simulink model "sampleModel1922"  (R2023a)
settings: Solver=VariableStepAuto  StartTime=0.0  StopTime=10.0  RelTol=1e-3
libraries: hdlsllib x6, simulink x1
settings Model: Creator=user1  LastModifiedBy=user1

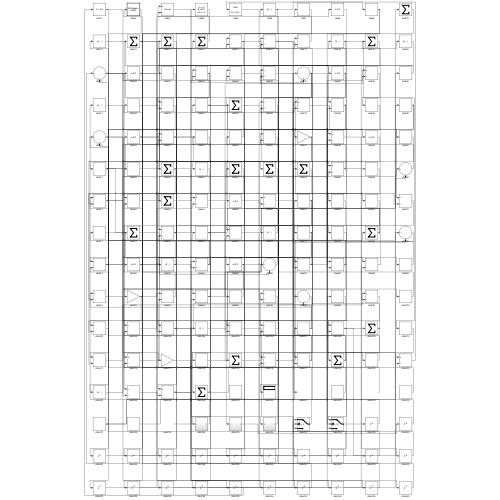
[thumbnail: Simulink's stored preview of the top-level diagram]
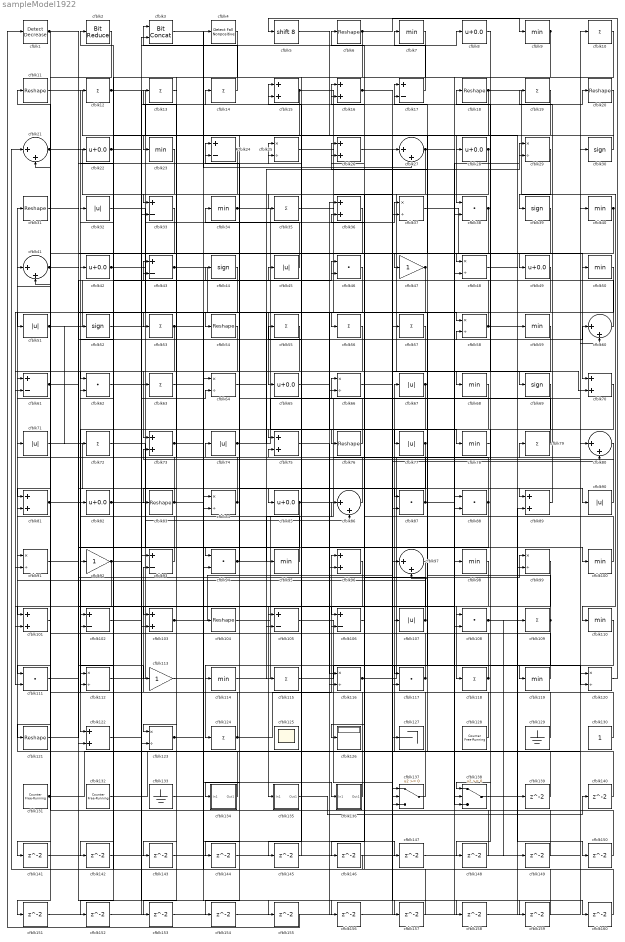
== system sampleModel1922 ==
  cfblk1 : simulink/Logic and Bit Operations/Detect Decrease  vinit=0.0  OutDataTypeStr=boolean
      settings: LibrarySourceBlock=|
      | hdlsllib/Logic and Bit
      | Operations/Detect
      | Decrease
  cfblk{10,12..14,19,35,53,55..57,63,72,79,109,115,118,124} (17 alike) : Sum  Inputs=+
  cfblk{7,9,23,34,40,50,59,68,78,95,98,100,110,114,119} (15 alike) : MinMax
  cfblk{15..16,26,36,70,73,75,81,89,96,101,103,122} (13 alike) : Sum
  cfblk{17,24,33,43,61,93,102,105..106} (9 alike) : Sum  Inputs=+-
  cfblk{6,11,18,20,31,54,76,83,104,121} (10 alike) : Reshape
  cfblk{32,45,51,67,71,74,77,90,107} (9 alike) : Abs  SaturateOnIntegerOverflow=off
  cfblk{38,46,62,87..88,94,108,111,117} (9 alike) : DotProduct  OutDataTypeStr=Inherit: Inherit via internal rule
  cfblk{25,29,37,48,58,64,66,84,91,99,112,116,120,123} (14 alike) : Product  Inputs=*/  RndMeth=Zero  SaturateOnIntegerOverflow=on
  cfblk113 : Gain
  cfblk125 : Scope
      settings: Floating=on
  cfblk126 : Display
  cfblk127 : Terminator
  cfblk128 : hdlsllib/Sources/Counter Free-Running  NumBits=16  tsamp=-1
  cfblk129 : Ground
  cfblk130 : Constant  SampleTime=-1
  cfblk131 : hdlsllib/Sources/Counter Free-Running  NumBits=16  tsamp=-1
  cfblk132 : hdlsllib/Sources/Counter Free-Running  NumBits=16  tsamp=-1
  cfblk133 : Ground
  cfblk134 : Subsystem
      settings: LibrarySourceBlock=|
      | hdlsllib/Ports &
      | Subsystems/Subsystem
  cfblk135 : Subsystem
      settings: LibrarySourceBlock=|
      | hdlsllib/Ports &
      | Subsystems/Subsystem
  cfblk136 : Subsystem
      settings: LibrarySourceBlock=|
      | hdlsllib/Ports &
      | Subsystems/Subsystem
  cfblk137 : Switch  SaturateOnIntegerOverflow=off  InputSameDT=off
  cfblk138 : Switch  SaturateOnIntegerOverflow=off  InputSameDT=off
  cfblk{139..160} (22 alike) : Delay  SampleTime=1
  cfblk2 : hdlsllib/Logic and Bit Operations/Bit Reduce  mode=AND
  cfblk{21,27,41,60,80,86,97} (7 alike) : Sum  Inputs=|++
  cfblk{8,22,28,42,49,65,82,85} (8 alike) : Bias  Bias=0.0  SaturateOnIntegerOverflow=off
  cfblk3 : hdlsllib/Logic and Bit Operations/Bit Concat  numInputs=2
  cfblk{30,39,44,52,69} (5 alike) : Signum
  cfblk4 : hdlsllib/Logic and Bit Operations/Detect Fall Nonpositive  vinit=0  OutDataTypeStr=boolean
  cfblk47 : Gain
  cfblk5 : ArithShift  BitShiftNumber=8
  cfblk92 : Gain
  wires:
  cfblk34/1 -> cfblk78/1, cfblk48/1
  cfblk77/1 -> cfblk85/1, cfblk134/1(In1)
  cfblk40/1 -> cfblk70/1, cfblk138/3
  cfblk134/1(Out1) -> cfblk31/1
  cfblk11/1 -> cfblk38/1
  cfblk76/1 -> cfblk66/1
  cfblk109/1 -> cfblk26/1, cfblk148/1
  cfblk124/1 -> cfblk96/1, cfblk11/1
  cfblk112/1 -> cfblk14/1
  cfblk115/1 -> cfblk119/1
  cfblk37/1 -> cfblk49/1
  cfblk95/1 -> cfblk12/1
  cfblk132/1 -> cfblk67/1
  cfblk27/1 -> cfblk70/2, cfblk120/2, cfblk35/1, cfblk153/1
  cfblk73/1 -> cfblk4/1, cfblk13/1
  cfblk26/1 -> cfblk69/1
  cfblk116/1 -> cfblk79/1, cfblk16/2
  cfblk67/1 -> cfblk122/1, cfblk105/2, cfblk97/2
  cfblk1/1 -> cfblk51/1, cfblk87/2
  cfblk129/1 -> cfblk42/1
  cfblk119/1 -> cfblk107/1
  cfblk105/1 -> cfblk137/3
  cfblk52/1 -> cfblk17/1
  cfblk96/1 -> cfblk135/1(In1)
  cfblk4/1 -> cfblk92/1
  cfblk108/1 -> cfblk149/1, cfblk150/1
  cfblk58/1 -> cfblk59/1, cfblk25/2
  cfblk39/1 -> cfblk101/1
  cfblk117/1 -> cfblk15/1, cfblk26/2
  cfblk53/1 -> cfblk91/2, cfblk155/1
  cfblk2/1 -> cfblk111/1
  cfblk41/1 -> cfblk54/1, cfblk100/1
  cfblk15/1 -> cfblk58/1, cfblk152/1
  cfblk136/1(Out1) -> cfblk32/1
  cfblk42/1 -> cfblk37/1, cfblk117/2
  cfblk6/1 -> cfblk62/1, cfblk9/1
  cfblk121/1 -> cfblk82/1
  cfblk18/1 -> cfblk110/1, cfblk154/1
  cfblk75/1 -> cfblk116/1
  cfblk104/1 -> cfblk57/1
  cfblk47/1 -> cfblk65/1, cfblk61/2
  cfblk61/1 -> cfblk58/2, cfblk113/1
  cfblk51/1 -> cfblk46/1, cfblk72/1, cfblk56/1
  cfblk14/1 -> cfblk3/1
  cfblk38/1 -> cfblk106/1, cfblk141/1
  cfblk101/1 -> cfblk121/1
  cfblk29/1 -> cfblk39/1
  cfblk35/1 -> cfblk88/1
  cfblk107/1 -> cfblk36/2, cfblk91/1
  cfblk63/1 -> cfblk25/1
  cfblk130/1 -> cfblk62/2
  cfblk114/1 -> cfblk40/1
  cfblk68/1 -> cfblk126/1
  cfblk79/1 -> cfblk45/1, cfblk24/1
  cfblk9/1 -> cfblk112/1, cfblk138/2
  cfblk19/1 -> cfblk47/1
  cfblk106/1 -> cfblk6/1
  cfblk36/1 -> cfblk105/1
  cfblk82/1 -> cfblk89/1, cfblk86/2
  cfblk62/1 -> cfblk60/1
  cfblk25/1 -> cfblk127/1
  cfblk137/1 -> cfblk93/2
  cfblk90/1 -> cfblk18/1
  cfblk72/1 -> cfblk94/1
  cfblk98/1 -> cfblk118/1
  cfblk46/1 -> cfblk81/1
  cfblk28/1 -> cfblk76/1, cfblk88/2
  cfblk85/1 -> cfblk30/1, cfblk122/2
  cfblk20/1 -> cfblk123/1
  cfblk120/1 -> cfblk5/1
  cfblk84/1 -> cfblk41/2, cfblk43/1
  cfblk103/1 -> cfblk37/2, cfblk156/1
  cfblk110/1 -> cfblk124/1
  cfblk64/1 -> cfblk115/1
  cfblk48/1 -> cfblk90/1
  cfblk30/1 -> cfblk23/1
  cfblk93/1 -> cfblk52/1
  cfblk71/1 -> cfblk109/1
  cfblk17/1 -> cfblk7/1
  cfblk21/1 -> cfblk123/2, cfblk24/2, cfblk50/1
  cfblk69/1 -> cfblk108/1
  cfblk49/1 -> cfblk53/1
  cfblk10/1 -> cfblk103/1
  cfblk43/1 -> cfblk66/2, cfblk20/1
  cfblk3/1 -> cfblk27/2
  cfblk74/1 -> cfblk60/2, cfblk29/2
  cfblk91/1 -> cfblk108/2
  cfblk111/1 -> cfblk99/1
  cfblk8/1 -> cfblk68/1
  cfblk65/1 -> cfblk77/1
  cfblk55/1 -> cfblk114/1
  cfblk128/1 -> cfblk112/2
  cfblk32/1 -> cfblk95/1
  cfblk7/1 -> cfblk75/1
  cfblk22/1 -> cfblk15/2, cfblk96/2
  cfblk81/1 -> cfblk87/1, cfblk43/2
  cfblk78/1 -> cfblk138/1
  cfblk89/1 -> cfblk19/1
  cfblk83/1 -> cfblk71/1, cfblk136/1(In1)
  cfblk23/1 -> cfblk103/2
  cfblk87/1 -> cfblk44/1, cfblk29/1
  cfblk86/1 -> cfblk61/1
  cfblk88/1 -> cfblk55/1, cfblk21/2, cfblk145/1
  cfblk50/1 -> cfblk117/1
  cfblk54/1 -> cfblk102/1
  cfblk118/1 -> cfblk22/1, cfblk81/2
  cfblk102/1 -> cfblk64/2
  cfblk100/1 -> cfblk16/1
  cfblk123/1 -> cfblk104/1, cfblk147/1
  cfblk131/1 -> cfblk98/1, cfblk10/1
  cfblk13/1 -> cfblk33/1
  cfblk59/1 -> cfblk111/2
  cfblk94/1 -> cfblk74/1, cfblk86/1
  cfblk56/1 -> cfblk73/1
  cfblk24/1 -> cfblk63/1, cfblk83/1
  cfblk66/1 -> cfblk97/1
  cfblk133/1 -> cfblk94/2
  cfblk12/1 -> cfblk33/2, cfblk99/2
  cfblk92/1 -> cfblk8/1, cfblk101/2
  cfblk44/1 -> cfblk84/2
  cfblk80/1 -> cfblk73/2
  cfblk5/1 -> cfblk28/1
  cfblk45/1 -> cfblk34/1
  cfblk16/1 -> cfblk80/2, cfblk160/1
  cfblk60/1 -> cfblk2/1
  cfblk138/1 -> cfblk139/1
  cfblk139/1 -> cfblk17/2
  cfblk135/1(Out1) -> cfblk140/1
  cfblk140/1 -> cfblk84/1
  cfblk141/1 -> cfblk36/1
  cfblk99/1 -> cfblk142/1
  cfblk142/1 -> cfblk93/1
  cfblk70/1 -> cfblk143/1
  cfblk143/1 -> cfblk137/2
  cfblk97/1 -> cfblk144/1
  cfblk144/1 -> cfblk120/1
  cfblk145/1 -> cfblk75/2
  cfblk57/1 -> cfblk146/1
  cfblk146/1 -> cfblk21/1
  cfblk147/1 -> cfblk38/2
  cfblk148/1 -> cfblk137/1
  cfblk149/1 -> cfblk41/1
  cfblk150/1 -> cfblk106/2
  cfblk33/1 -> cfblk151/1
  cfblk151/1 -> cfblk27/1
  cfblk152/1 -> cfblk3/2
  cfblk153/1 -> cfblk48/2
  cfblk154/1 -> cfblk116/2
  cfblk155/1 -> cfblk1/1
  cfblk156/1 -> cfblk89/2
  cfblk122/1 -> cfblk157/1
  cfblk157/1 -> cfblk46/2
  cfblk31/1 -> cfblk158/1
  cfblk158/1 -> cfblk80/1
  cfblk113/1 -> cfblk159/1
  cfblk159/1 -> cfblk64/1
  cfblk160/1 -> cfblk102/2

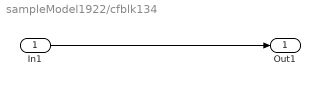
== system sampleModel1922/cfblk134 ==
  In1 : Inport
  Out1 : Outport
  wires:
  In1/1 -> Out1/1

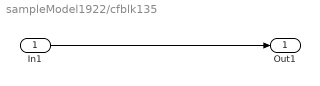
== system sampleModel1922/cfblk135 ==
  In1 : Inport
  Out1 : Outport
  wires:
  In1/1 -> Out1/1

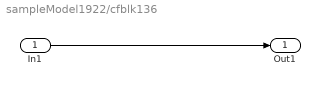
== system sampleModel1922/cfblk136 ==
  In1 : Inport
  Out1 : Outport
  wires:
  In1/1 -> Out1/1
